simulink model "BlanceCar"  (R2018b)
settings: Solver=FixedStepDiscrete  StartTime=0.0  StopTime=10  FixedStep=0.001  RelTol=1e-3  EnableMultiTasking=on
libraries: mylib x4
settings Model: Creator=Gavin  LastModifiedBy=Gavin
settings OptimizationCC: DefaultParameterBehavior=Inlined  EnhancedBackFolding=on  PassReuseOutputArgsAs=Individual arguments  OptimizeBlockOrder=speed  DifferentSizesBufferReuse=on  OptimizationCustomize=off
settings DebuggingCC: ParameterTunabilityLossMsg=error
settings HardwareCC: ProdBitPerPointer=32  ProdBitPerSizeT=32  ProdBitPerPtrDiffT=32  ProdLargestAtomicInteger=Long  ProdLargestAtomicFloat=Double  ProdWordSize=32  ProdHWDeviceType=ARM Compatible->ARM Cortex
settings SFSimCC: MATLABDynamicMemAlloc=off
settings RTWCC: SystemTargetFile=ert.tlc  TemplateMakefile=ert_default_tmf  GenerateReport=on  IncludeHyperlinkInReport=on  LaunchReport=on  GenerateTraceInfo=on  GenerateTraceReport=on  GenerateTraceReportSl=on  GenerateTraceReportSf=on  GenerateTraceReportEml=on
settings CodeAppCC: ForceParamTrailComments=on  IgnoreCustomStorageClasses=off  OperatorAnnotations=on  SimulinkDataObjDesc=on  SFDataObjDesc=on  InsertBlockDesc=on
settings ERTTargetCC: TargetLangStandard=C99 (ISO)  GenerateSampleERTMain=on  InlinedParameterPlacement=NonHierarchical  ERTCustomFileTemplate=example_file_process.tlc

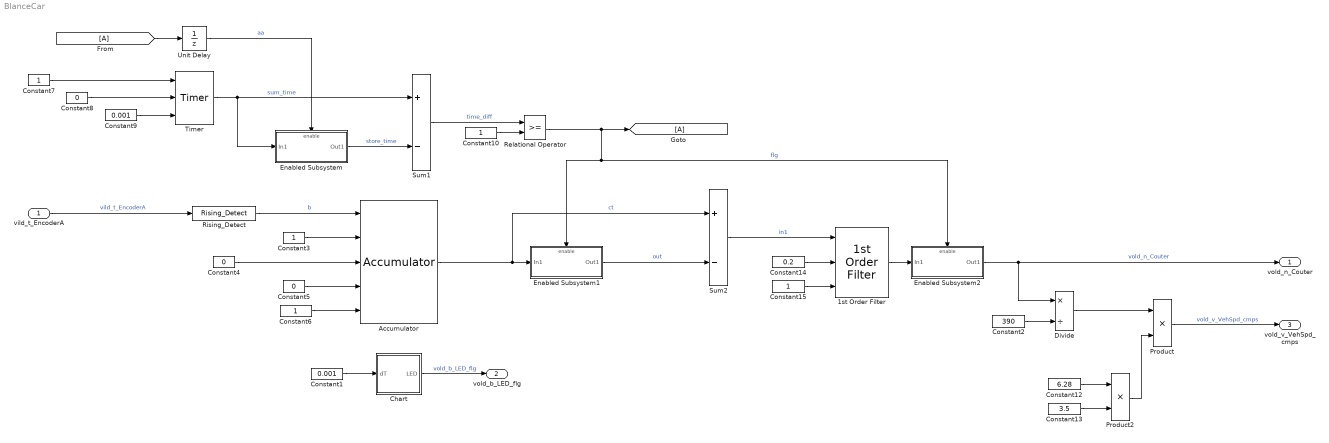
== system BlanceCar ==
  vild_t_EncoderA : Inport
  1st Order Filter : mylib/Filters/1st Order Filter  SystemSampleTime=-1
  Accumulator : mylib/Intergrators/Accumulator  InitValue=0
  Chart : Stateflow chart  TreatAsAtomicUnit=on
  Constant1 : Constant  Value=0.001  OutDataTypeStr=single  SampleTime=-1
      settings: AttributesFormatString=<%<OutDataTypeStr>>
  Constant10 : Constant  OutDataTypeStr=single  SampleTime=-1
      settings: AttributesFormatString=<%<OutDataTypeStr>>
  Constant12 : Constant  Value=6.28  OutDataTypeStr=single  SampleTime=-1
      settings: AttributesFormatString=<%<OutDataTypeStr>>
  Constant13 : Constant  Value=3.5  OutDataTypeStr=single  SampleTime=-1
      settings: AttributesFormatString=<%<OutDataTypeStr>>
  Constant14 : Constant  Value=0.2  OutDataTypeStr=single  SampleTime=-1
      settings: AttributesFormatString=<%<OutDataTypeStr>>
  Constant15 : Constant  OutDataTypeStr=single  SampleTime=-1
      settings: AttributesFormatString=<%<OutDataTypeStr>>
  Constant2 : Constant  Value=390  OutDataTypeStr=single  SampleTime=-1
      settings: AttributesFormatString=<%<OutDataTypeStr>>
  Constant3 : Constant  OutDataTypeStr=boolean  SampleTime=-1
      settings: AttributesFormatString=<%<OutDataTypeStr>>
  Constant4 : Constant  Value=0  OutDataTypeStr=boolean  SampleTime=-1
      settings: AttributesFormatString=<%<OutDataTypeStr>>
  Constant5 : Constant  Value=0  OutDataTypeStr=single  SampleTime=-1
      settings: AttributesFormatString=<%<OutDataTypeStr>>
  Constant6 : Constant  OutDataTypeStr=single  SampleTime=-1
      settings: AttributesFormatString=<%<OutDataTypeStr>>
  Constant7 : Constant  OutDataTypeStr=boolean  SampleTime=-1
      settings: AttributesFormatString=<%<OutDataTypeStr>>
  Constant8 : Constant  Value=0  OutDataTypeStr=boolean  SampleTime=-1
      settings: AttributesFormatString=<%<OutDataTypeStr>>
  Constant9 : Constant  Value=0.001  OutDataTypeStr=single  SampleTime=-1
      settings: AttributesFormatString=<%<OutDataTypeStr>>
  Divide : Product  Inputs=*/
  Enabled Subsystem : Subsystem  TreatAsAtomicUnit=on
  Enabled Subsystem1 : Subsystem  TreatAsAtomicUnit=on
  Enabled Subsystem2 : Subsystem  TreatAsAtomicUnit=on
  Product : Product  RndMeth=Zero
  Product2 : Product  RndMeth=Zero
  Relational Operator : RelationalOperator  OutDataTypeStr=boolean  RndMeth=Nearest
  Rising_Detect : mylib/Memory/Rising_Detect  SystemSampleTime=-1
  Sum1 : Sum  Inputs=+-  RndMeth=Zero
  Sum2 : Sum  Inputs=+-  RndMeth=Zero
  Timer : mylib/Counter&Timer/Timer  SystemSampleTime=-1
  Unit Delay : UnitDelay  SampleTime=-1
      settings: AttributesFormatString=<initial=%<x0>>
  vold_n_Couter : Outport
  vold_b_LED_flg : Outport  Port=2
  vold_v_VehSpd_cmps : Outport  Port=3
  wires:
  Constant7/1 -> Timer/1
  Constant8/1 -> Timer/2
  Constant9/1 -> Timer/3
  Timer/1 -> Enabled Subsystem/1(In1), Sum1/1  "sum_time"
  Enabled Subsystem/1(Out1) -> Sum1/2  "store_time"
  Constant10/1 -> Relational Operator/2
  Relational Operator/1 -> [A], Enabled Subsystem2/Enable, Enabled Subsystem1/Enable  "flg"
  Enabled Subsystem2/1(Out1) -> Divide/1, vold_n_Couter/1  "vold_n_Couter"
  Unit Delay/1 -> Enabled Subsystem/Enable  "aa"
  [A] -> Unit Delay/1
  Sum1/1 -> Relational Operator/1  "time_diff"
  Rising_Detect/1 -> Accumulator/1  "b"
  Constant6/1 -> Accumulator/5
  Constant4/1 -> Accumulator/3
  Constant3/1 -> Accumulator/2
  Constant5/1 -> Accumulator/4
  Accumulator/1 -> Sum2/1, Enabled Subsystem1/1(In1)  "ct"
  Constant1/1 -> Chart/1(dT)
  Chart/1(LED) -> vold_b_LED_flg/1  "vold_b_LED_flg"
  Enabled Subsystem1/1(Out1) -> Sum2/2  "out"
  Sum2/1 -> 1st Order Filter/1  "in1"
  vild_t_EncoderA/1 -> Rising_Detect/1  "vild_t_EncoderA"
  Constant2/1 -> Divide/2
  Divide/1 -> Product/1
  Constant12/1 -> Product2/1
  Constant13/1 -> Product2/2
  Product2/1 -> Product/2
  Product/1 -> vold_v_VehSpd_cmps/1  "vold_v_VehSpd_cmps"
  1st Order Filter/1 -> Enabled Subsystem2/1(In1)
  Constant14/1 -> 1st Order Filter/2
  Constant15/1 -> 1st Order Filter/3

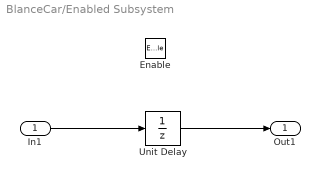
== system BlanceCar/Enabled Subsystem ==
  In1 : Inport
  Enable : EnablePort
  Unit Delay : UnitDelay  InitialCondition=-1  SampleTime=-1
  Out1 : Outport
  wires:
  In1/1 -> Unit Delay/1
  Unit Delay/1 -> Out1/1

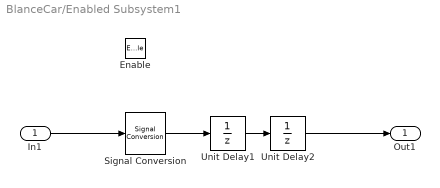
== system BlanceCar/Enabled Subsystem1 ==
  In1 : Inport
  Enable : EnablePort
  Signal Conversion : SignalConversion  OverrideOpt=off
  Unit Delay1 : UnitDelay  SampleTime=-1
      settings: AttributesFormatString=<initial=%<x0>>
  Unit Delay2 : UnitDelay  SampleTime=-1
      settings: AttributesFormatString=<initial=%<x0>>
  Out1 : Outport
  wires:
  In1/1 -> Signal Conversion/1
  Signal Conversion/1 -> Unit Delay1/1
  Unit Delay1/1 -> Unit Delay2/1
  Unit Delay2/1 -> Out1/1

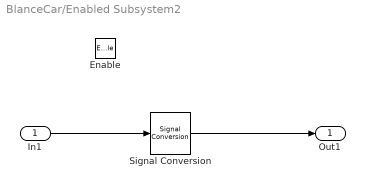
== system BlanceCar/Enabled Subsystem2 ==
  In1 : Inport
  Enable : EnablePort
  Signal Conversion : SignalConversion  OverrideOpt=off
  Out1 : Outport
  wires:
  In1/1 -> Signal Conversion/1
  Signal Conversion/1 -> Out1/1

== stateflow chart BlanceCar/Chart ==
  settings: executeAtInitialization=1  enableNonTerminalStates=1
  state LED_ON
    en:
    LED = 0;
    timer = 0;
    du:
    timer=timer+dT;
  state LED_OFF
    en:
    LED = 1;
    timer = 0;
    du:
    timer = timer+dT;
  (default) -> LED_ON
  LED_ON -> LED_OFF : [timer>=0.5]
  LED_OFF -> LED_ON : [timer>=0.5]
  data: LED output boolean; timer local single; dT input single
